simulink model "HW_7_2_system"  (R2017a)
settings: Solver=VariableStepAuto  StartTime=0.0  StopTime=50  RelTol=1e-3  EnableMultiTasking=on
settings Model: Creator=Teng-Hu  LastModifiedBy=USER
settings OptimizationCC: LifeSpan=inf
settings DebuggingCC: SFUnexpectedBacktrackingDiag=warning  SFNoUnconditionalDefaultTransitionDiag=warning  SFExecutionAtInitializationDiag=none
settings GRTTargetCC: TargetLangStandard=C89/C90 (ANSI)
settings ConfigComp: CovMetricSettings=dw  CovHtmlReporting=on  CovSaveCumulativeToWorkspaceVar=on  CovSaveSingleToWorkspaceVar=on  CovExternalEMLEnable=off

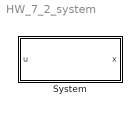
== system HW_7_2_system ==
  System : Subsystem

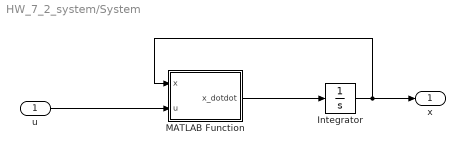
== system HW_7_2_system/System ==
  u : Inport
  Integrator : Integrator  InitialCondition=1
  MATLAB Function : MATLAB Function  TreatAsAtomicUnit=on
  x : Outport
  wires:
  Integrator/1 -> MATLAB Function/1(x), x/1
  u/1 -> MATLAB Function/2(u)
  MATLAB Function/1(x_dotdot) -> Integrator/1

== matlab function HW_7_2_system/System/MATLAB Function ==
  data: x input; u input; x_dotdot output
function x_dotdot = fcn(x,u)
%#codegen

x_dotdot = 2*x+5*cos(x)+u;
